simulink model "Final2017"  (R2016a)
settings: Solver=VariableStepAuto  StartTime=0.0  StopTime=10  RelTol=1e-3
values from neighbouring files (symbols this model uses):
  A1 = -A(1,1)    [FInal2019.m]    (also in FInal_3_12_2021.m; Final2017.m; Final2018.m; Final2020feb.m)
  A2 = -A(1,2)    [FInal2019.m]    (also in FInal_3_12_2021.m; Final2017.m; Final2018.m; Final2020feb.m)
  A3 = -A(1,3)    [FInal2019.m]    (also in FInal_3_12_2021.m; Final2017.m; Final2018.m; Final2020feb.m)
  K1 = K(1,1)    [FInal2019.m]    (also in FInal_3_12_2021.m = khat(1,1); Final2017.m; Final2018.m; Final2020feb.m = khat(1,1))
  K2 = K(1,2)    [FInal2019.m]    (also in FInal_3_12_2021.m = khat(1,2); Final2017.m; Final2018.m; Final2020feb.m = khat(1,2))
  K3 = K(1,3)    [FInal2019.m]    (also in FInal_3_12_2021.m = khat(1,3); Final2017.m; Final2018.m; Final2020feb.m = khat(1,3))
libraries: simulink x1
settings Model: Creator=alber  LastModifiedBy=alber

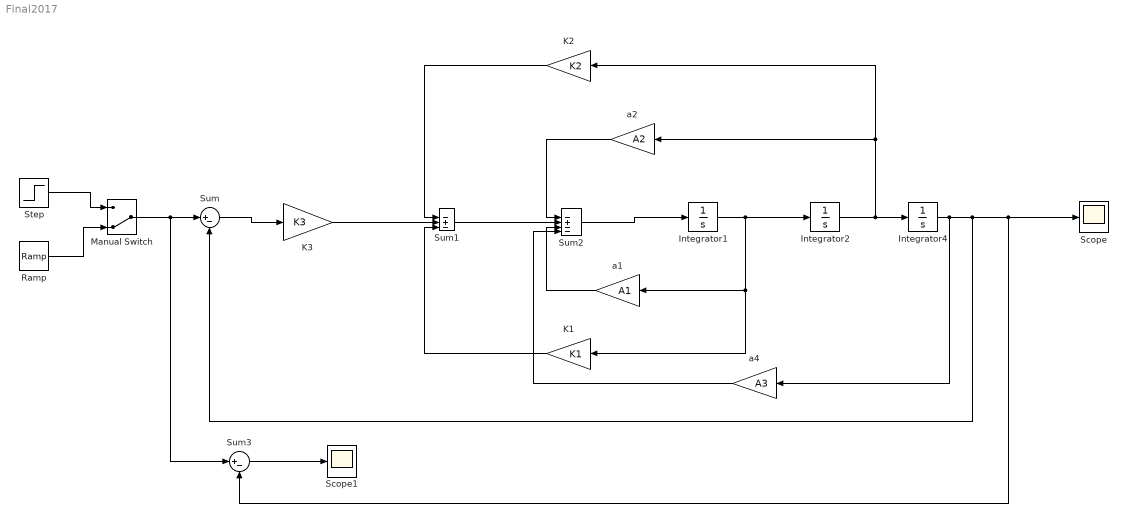
== system Final2017 ==
  Integrator1 : Integrator
  Integrator2 : Integrator
  Integrator4 : Integrator
  K1 : Gain  Gain=K1
  K2 : Gain  Gain=K2
  K3 : Gain  Gain=K3
  Manual Switch : ManualSwitch  CurrentSetting=0
  Ramp : simulink/Sources/Ramp  slope=1  start=0  X0=0
  Scope : Scope
  Scope1 : Scope
  Step : Step  SampleTime=0
  Sum : Sum  Inputs=|+-
  Sum1 : Sum  Inputs=|-+-
  Sum2 : Sum  Inputs=|-+--
  Sum3 : Sum  Inputs=|+-
  a1 : Gain  Gain=A1
  a2 : Gain  Gain=A2
  a4 : Gain  Gain=A3
  wires:
  Sum1/1 -> Sum2/2
  Sum2/1 -> Integrator1/1
  Integrator1/1 -> K1/1, a1/1, Integrator2/1
  a1/1 -> Sum2/3
  K1/1 -> Sum1/3
  a2/1 -> Sum2/1
  Sum/1 -> K3/1
  Integrator2/1 -> Integrator4/1, K2/1, a2/1
  Manual Switch/1 -> Sum3/1, Sum/1
  Step/1 -> Manual Switch/1
  Ramp/1 -> Manual Switch/2
  K3/1 -> Sum1/2
  K2/1 -> Sum1/1
  Sum3/1 -> Scope1/1
  a4/1 -> Sum2/4
  Integrator4/1 -> a4/1, Sum3/2, Scope/1, Sum/2
